simulink model "BigFourStEnCtrl"  (R2018b)
settings: Solver=FixedStepDiscrete  StartTime=0.0  StopTime=10.0  FixedStep=0.01  RelTol=1e-3
undefined symbols (not defined in the file or in its folder): data, KeSMSw4SSecRwLtStLgrstOtwdInwdClosePos1_Val, KeSMSw4SSecRwLtStLgrstUpwdDnwdClosePos1_Val, KeSMSw4SSecRwLtStLgrstUpwdDnwdClosePos2_Val, PassStBkReclnEn_Clear, PassStBkReclnEn_Set, PassStFwdBkwdEn_Clear, PassStFwdBkwdEn_Set, SecRwLtStBkReclnEn_Clear, SecRwLtStBkReclnEn_Set, SecRwLtStFwdBkwdEn_Clear, SecRwLtStFwdBkwdEn_Set, SecRwLtStLgrstInwdOtwdEn_Clear, SecRwLtStLgrstInwdOtwdEn_Set, SecRwLtStLgrstUpwdDnwdEn_Clear, SecRwLtStLgrstUpwdDnwdEn_Set, SecRwRtStBkReclnEn_Clear, SecRwRtStBkReclnEn_Set, SecRwRtStFwdBkwdEn_Clear, SecRwRtStFwdBkwdEn_Set, SecRwRtStLgrstInwdOtwdEn_Clear, SecRwRtStLgrstInwdOtwdEn_Set, SecRwRtStLgrstUpwdDnwdEn_Clear, SecRwRtStLgrstUpwdDnwdEn_Set, ThdRwLtStBkReclnEn_Clear, ThdRwLtStBkReclnEn_Set, ThdRwLtStCshnFldEn_Clear, ThdRwLtStCshnFldEn_Set, ThdRwLtStFwdBkwdEn_Clear, ThdRwLtStFwdBkwdEn_Set, ThdRwRtStBkReclnEn_Clear, ThdRwRtStBkReclnEn_Set, ThdRwRtStCshnFldEn_Clear, ThdRwRtStCshnFldEn_Set, ThdRwRtStFwdBkwdEn_Clear, ThdRwRtStFwdBkwdEn_Set, ZeroLEn_Clear, ZeroLEn_Set, ZeroREn_Clear, ZeroREn_Set
libraries: simulink x1
(part 1 of 2)
settings Model: Creator=sn2xws  LastModifiedBy=sn55gm
settings Model: ModifiedHistory=|
  | 2024.9.9 新增Md56
  | 2024.9.26 V3.0.1 从Md1V3.0.4复制
  | 2024.11.12 V3.0.2 Md1 bug 945653问题同步
settings DataIOCC: SaveFormat=StructureWithTime
settings OptimizationCC: DefaultParameterBehavior=Inlined  EnhancedBackFolding=on  PassReuseOutputArgsAs=Individual arguments  ZeroExternalMemoryAtStartup=off  ZeroInternalMemoryAtStartup=off  OptimizeBlockOrder=speed  DifferentSizesBufferReuse=on  OptimizationCustomize=off
settings DebuggingCC: ParameterTunabilityLossMsg=error
settings SFSimCC: MATLABDynamicMemAlloc=off
settings RTWCC: SystemTargetFile=autosar.tlc  GenCodeOnly=on  TemplateMakefile=ert_default_tmf  Description=AUTOSAR  GenerateReport=on  IncludeHyperlinkInReport=on  LaunchReport=on  GenerateTraceInfo=on  GenerateTraceReport=on  GenerateTraceReportSl=on  GenerateTraceReportSf=on  GenerateTraceReportEml=on
settings CodeAppCC: ForceParamTrailComments=on  IgnoreCustomStorageClasses=off  OperatorAnnotations=on  SimulinkDataObjDesc=on  SFDataObjDesc=on  InsertBlockDesc=on
settings STFCustomTargetCC: TargetLangStandard=C99 (ISO)  MultiwordLength=256  ParMdlRefBuildCompliant=on  CompOptLevelCompliant=on  IncludeMdlTerminateFcn=off  CombineOutputUpdateFcns=on  SuppressErrorStatus=on  ERTCustomFileBanners=on  SupportNonFinite=off  SupportComplex=off  SupportContinuousTime=off  SupportNonInlinedSFcns=off  RemoveResetFunc=on  MATLABClassNameForMDSCustomization=Simulink.SoftwareTarget.ERTCustomization  AutosarCompliant=on  UseToolchainInfoCompliant=on  LookupTableObjectStructAxisOrder=2,1,3,4,...  LUTObjectStructOrderEvenSpacing=Size,Table,Breakpoints  SystemTargetFile=autosar.tlc
settings ERTTargetCC: TargetLangStandard=C99 (ISO)  ConcurrentExecutionCompliant=off  IncludeMdlTerminateFcn=off  SuppressErrorStatus=on  SupportNonFinite=off  SupportComplex=off  ModelStepFunctionPrototypeControlCompliant=off  CPPClassGenCompliant=off  AutosarCompliant=on  LookupTableObjectStructAxisOrder=2,1,3,4,...  LUTObjectStructOrderEvenSpacing=Size,Table,Breakpoints  InlinedParameterPlacement=NonHierarchical  ERTCustomFileTemplate=example_file_process.tlc  ERTFilePackagingFormat=Compact  BooleanTrueId=TRUE  BooleanFalseId=FALSE

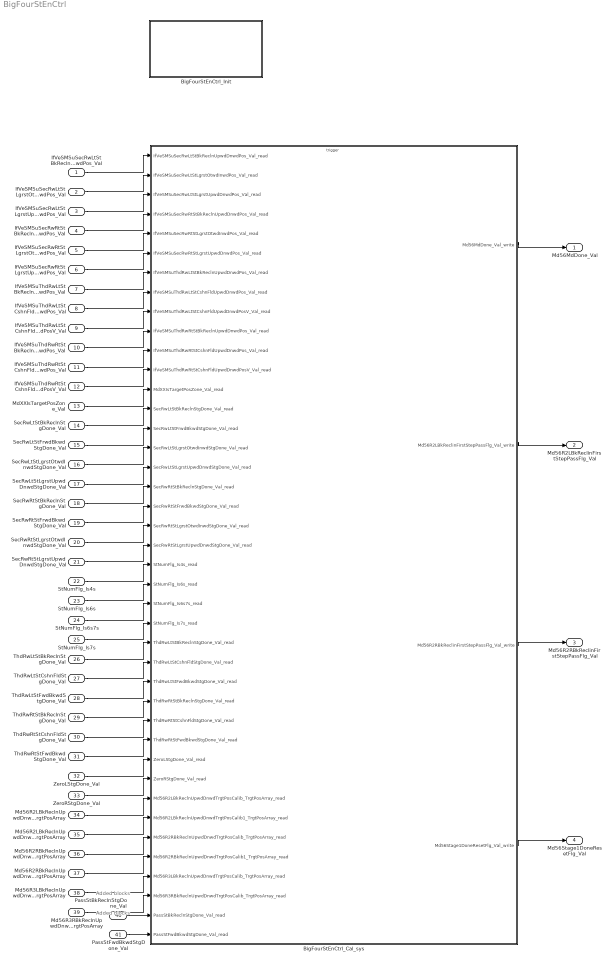
== system BigFourStEnCtrl ==
  note: Added blocks
  note: Added blocks
  IfVeSMSuSecRwLtStBkReclnUpwdDnwdPos_Val : Inport  OutDataTypeStr=uint16  PortDimensions=1
  IfVeSMSuSecRwLtStLgrstOtwdInwdPos_Val : Inport  Port=2  OutDataTypeStr=uint16  PortDimensions=1
  IfVeSMSuSecRwLtStLgrstUpwdDnwdPos_Val : Inport  Port=3  OutDataTypeStr=uint16  PortDimensions=1
  IfVeSMSuSecRwRtStBkReclnUpwdDnwdPos_Val : Inport  Port=4  OutDataTypeStr=uint16  PortDimensions=1
  IfVeSMSuSecRwRtStLgrstOtwdInwdPos_Val : Inport  Port=5  OutDataTypeStr=uint16  PortDimensions=1
  IfVeSMSuSecRwRtStLgrstUpwdDnwdPos_Val : Inport  Port=6  OutDataTypeStr=uint16  PortDimensions=1
  IfVeSMSuThdRwLtStBkReclnUpwdDnwdPos_Val : Inport  Port=7  OutDataTypeStr=uint16  PortDimensions=1
  IfVeSMSuThdRwLtStCshnFldUpwdDnwdPos_Val : Inport  Port=8  OutDataTypeStr=uint16  PortDimensions=1
  IfVeSMSuThdRwLtStCshnFldUpwdDnwdPosV_Val : Inport  Port=9  OutDataTypeStr=boolean  PortDimensions=1
  IfVeSMSuThdRwRtStBkReclnUpwdDnwdPos_Val : Inport  Port=10  OutDataTypeStr=uint16  PortDimensions=1
  IfVeSMSuThdRwRtStCshnFldUpwdDnwdPos_Val : Inport  Port=11  OutDataTypeStr=uint16  PortDimensions=1
  IfVeSMSuThdRwRtStCshnFldUpwdDnwdPosV_Val : Inport  Port=12  OutDataTypeStr=boolean  PortDimensions=1
  MdXXIsTargetPosZone_Val : Inport  Port=13  OutDataTypeStr=uint32  PortDimensions=1
  SecRwLtStBkReclnStgDone_Val : Inport  Port=14  OutDataTypeStr=boolean  PortDimensions=1
  SecRwLtStFrwdBkwdStgDone_Val : Inport  Port=15  OutDataTypeStr=boolean  PortDimensions=1
  SecRwLtStLgrstOtwdInwdStgDone_Val : Inport  Port=16  OutDataTypeStr=boolean  PortDimensions=1
  SecRwLtStLgrstUpwdDnwdStgDone_Val : Inport  Port=17  OutDataTypeStr=boolean  PortDimensions=1
  SecRwRtStBkReclnStgDone_Val : Inport  Port=18  OutDataTypeStr=boolean  PortDimensions=1
  SecRwRtStFrwdBkwdStgDone_Val : Inport  Port=19  OutDataTypeStr=boolean  PortDimensions=1
  SecRwRtStLgrstOtwdInwdStgDone_Val : Inport  Port=20  OutDataTypeStr=boolean  PortDimensions=1
  SecRwRtStLgrstUpwdDnwdStgDone_Val : Inport  Port=21  OutDataTypeStr=boolean  PortDimensions=1
  StNumFlg_Is4s : Inport  Port=22  OutDataTypeStr=boolean  PortDimensions=1
  StNumFlg_Is6s : Inport  Port=23  OutDataTypeStr=boolean  PortDimensions=1
  StNumFlg_Is6s7s : Inport  Port=24  OutDataTypeStr=boolean  PortDimensions=1
  StNumFlg_Is7s : Inport  Port=25  OutDataTypeStr=boolean  PortDimensions=1
  ThdRwLtStBkReclnStgDone_Val : Inport  Port=26  OutDataTypeStr=boolean  PortDimensions=1
  ThdRwLtStCshnFldStgDone_Val : Inport  Port=27  OutDataTypeStr=boolean  PortDimensions=1
  ThdRwLtStFwdBkwdStgDone_Val : Inport  Port=28  OutDataTypeStr=boolean  PortDimensions=1
  ThdRwRtStBkReclnStgDone_Val : Inport  Port=29  OutDataTypeStr=boolean  PortDimensions=1
  ThdRwRtStCshnFldStgDone_Val : Inport  Port=30  OutDataTypeStr=boolean  PortDimensions=1
  ThdRwRtStFwdBkwdStgDone_Val : Inport  Port=31  OutDataTypeStr=boolean  PortDimensions=1
  ZeroLStgDone_Val : Inport  Port=32  OutDataTypeStr=boolean  PortDimensions=1
  ZeroRStgDone_Val : Inport  Port=33  OutDataTypeStr=boolean  PortDimensions=1
  Md56R2LBkReclnUpwdDnwdTrgtPosCalib_TrgtPosArray : Inport  Description=|  Port=34  OutDataTypeStr=uint16  PortDimensions=3
      | 0:Pos
      | 1:Max
      | 2:Min
  Md56R2LBkReclnUpwdDnwdTrgtPosCalib1_TrgtPosArray : Inport  Description=|  Port=35  OutDataTypeStr=uint16  PortDimensions=3
      | 0:Pos
      | 1:Max
      | 2:Min
  Md56R2RBkReclnUpwdDnwdTrgtPosCalib_TrgtPosArray : Inport  Description=|  Port=36  OutDataTypeStr=uint16  PortDimensions=3
      | 0:Pos
      | 1:Max
      | 2:Min
  Md56R2RBkReclnUpwdDnwdTrgtPosCalib1_TrgtPosArray : Inport  Description=|  Port=37  OutDataTypeStr=uint16  PortDimensions=3
      | 0:Pos
      | 1:Max
      | 2:Min
  Md56R3LBkReclnUpwdDnwdTrgtPosCalib_TrgtPosArray : Inport  Description=|  Port=38  OutDataTypeStr=uint16  PortDimensions=3
      | 0:Pos
      | 1:Max
      | 2:Min
  Md56R3RBkReclnUpwdDnwdTrgtPosCalib_TrgtPosArray : Inport  Description=|  Port=39  OutDataTypeStr=uint16  PortDimensions=3
      | 0:Pos
      | 1:Max
      | 2:Min
  PassStBkReclnStgDone_Val : Inport  Port=40  OutDataTypeStr=boolean  PortDimensions=1
  PassStFwdBkwdStgDone_Val : Inport  Port=41  OutDataTypeStr=boolean  PortDimensions=1
  BigFourStEnCtrl_Cal_sys : Subsystem
  BigFourStEnCtrl_Init : Subsystem
  Md56MdDone_Val : Outport  OutDataTypeStr=uint8  PortDimensions=1
  Md56R2LBkReclinFirstStepPassFlg_Val : Outport  Port=2  OutDataTypeStr=boolean  PortDimensions=1
  Md56R2RBkReclinFirstStepPassFlg_Val : Outport  Port=3  OutDataTypeStr=boolean  PortDimensions=1
  Md56Stage1DoneResetFlg_Val : Outport  Port=4  OutDataTypeStr=boolean  PortDimensions=1
  wires:
  IfVeSMSuSecRwLtStBkReclnUpwdDnwdPos_Val/1 -> BigFourStEnCtrl_Cal_sys/1(IfVeSMSuSecRwLtStBkReclnUpwdDnwdPos_Val_read)
  IfVeSMSuSecRwLtStLgrstOtwdInwdPos_Val/1 -> BigFourStEnCtrl_Cal_sys/2(IfVeSMSuSecRwLtStLgrstOtwdInwdPos_Val_read)
  IfVeSMSuSecRwLtStLgrstUpwdDnwdPos_Val/1 -> BigFourStEnCtrl_Cal_sys/3(IfVeSMSuSecRwLtStLgrstUpwdDnwdPos_Val_read)
  IfVeSMSuSecRwRtStBkReclnUpwdDnwdPos_Val/1 -> BigFourStEnCtrl_Cal_sys/4(IfVeSMSuSecRwRtStBkReclnUpwdDnwdPos_Val_read)
  IfVeSMSuSecRwRtStLgrstOtwdInwdPos_Val/1 -> BigFourStEnCtrl_Cal_sys/5(IfVeSMSuSecRwRtStLgrstOtwdInwdPos_Val_read)
  IfVeSMSuSecRwRtStLgrstUpwdDnwdPos_Val/1 -> BigFourStEnCtrl_Cal_sys/6(IfVeSMSuSecRwRtStLgrstUpwdDnwdPos_Val_read)
  IfVeSMSuThdRwLtStBkReclnUpwdDnwdPos_Val/1 -> BigFourStEnCtrl_Cal_sys/7(IfVeSMSuThdRwLtStBkReclnUpwdDnwdPos_Val_read)
  IfVeSMSuThdRwLtStCshnFldUpwdDnwdPos_Val/1 -> BigFourStEnCtrl_Cal_sys/8(IfVeSMSuThdRwLtStCshnFldUpwdDnwdPos_Val_read)
  IfVeSMSuThdRwLtStCshnFldUpwdDnwdPosV_Val/1 -> BigFourStEnCtrl_Cal_sys/9(IfVeSMSuThdRwLtStCshnFldUpwdDnwdPosV_Val_read)
  IfVeSMSuThdRwRtStBkReclnUpwdDnwdPos_Val/1 -> BigFourStEnCtrl_Cal_sys/10(IfVeSMSuThdRwRtStBkReclnUpwdDnwdPos_Val_read)
  IfVeSMSuThdRwRtStCshnFldUpwdDnwdPos_Val/1 -> BigFourStEnCtrl_Cal_sys/11(IfVeSMSuThdRwRtStCshnFldUpwdDnwdPos_Val_read)
  IfVeSMSuThdRwRtStCshnFldUpwdDnwdPosV_Val/1 -> BigFourStEnCtrl_Cal_sys/12(IfVeSMSuThdRwRtStCshnFldUpwdDnwdPosV_Val_read)
  MdXXIsTargetPosZone_Val/1 -> BigFourStEnCtrl_Cal_sys/13(MdXXIsTargetPosZone_Val_read)
  SecRwLtStBkReclnStgDone_Val/1 -> BigFourStEnCtrl_Cal_sys/14(SecRwLtStBkReclnStgDone_Val_read)
  SecRwLtStFrwdBkwdStgDone_Val/1 -> BigFourStEnCtrl_Cal_sys/15(SecRwLtStFrwdBkwdStgDone_Val_read)
  SecRwLtStLgrstOtwdInwdStgDone_Val/1 -> BigFourStEnCtrl_Cal_sys/16(SecRwLtStLgrstOtwdInwdStgDone_Val_read)
  SecRwLtStLgrstUpwdDnwdStgDone_Val/1 -> BigFourStEnCtrl_Cal_sys/17(SecRwLtStLgrstUpwdDnwdStgDone_Val_read)
  SecRwRtStBkReclnStgDone_Val/1 -> BigFourStEnCtrl_Cal_sys/18(SecRwRtStBkReclnStgDone_Val_read)
  SecRwRtStFrwdBkwdStgDone_Val/1 -> BigFourStEnCtrl_Cal_sys/19(SecRwRtStFrwdBkwdStgDone_Val_read)
  SecRwRtStLgrstOtwdInwdStgDone_Val/1 -> BigFourStEnCtrl_Cal_sys/20(SecRwRtStLgrstOtwdInwdStgDone_Val_read)
  SecRwRtStLgrstUpwdDnwdStgDone_Val/1 -> BigFourStEnCtrl_Cal_sys/21(SecRwRtStLgrstUpwdDnwdStgDone_Val_read)
  StNumFlg_Is4s/1 -> BigFourStEnCtrl_Cal_sys/22(StNumFlg_Is4s_read)
  StNumFlg_Is6s/1 -> BigFourStEnCtrl_Cal_sys/23(StNumFlg_Is6s_read)
  StNumFlg_Is6s7s/1 -> BigFourStEnCtrl_Cal_sys/24(StNumFlg_Is6s7s_read)
  StNumFlg_Is7s/1 -> BigFourStEnCtrl_Cal_sys/25(StNumFlg_Is7s_read)
  ThdRwLtStBkReclnStgDone_Val/1 -> BigFourStEnCtrl_Cal_sys/26(ThdRwLtStBkReclnStgDone_Val_read)
  ThdRwLtStCshnFldStgDone_Val/1 -> BigFourStEnCtrl_Cal_sys/27(ThdRwLtStCshnFldStgDone_Val_read)
  ThdRwLtStFwdBkwdStgDone_Val/1 -> BigFourStEnCtrl_Cal_sys/28(ThdRwLtStFwdBkwdStgDone_Val_read)
  ThdRwRtStBkReclnStgDone_Val/1 -> BigFourStEnCtrl_Cal_sys/29(ThdRwRtStBkReclnStgDone_Val_read)
  ThdRwRtStCshnFldStgDone_Val/1 -> BigFourStEnCtrl_Cal_sys/30(ThdRwRtStCshnFldStgDone_Val_read)
  ThdRwRtStFwdBkwdStgDone_Val/1 -> BigFourStEnCtrl_Cal_sys/31(ThdRwRtStFwdBkwdStgDone_Val_read)
  ZeroLStgDone_Val/1 -> BigFourStEnCtrl_Cal_sys/32(ZeroLStgDone_Val_read)
  ZeroRStgDone_Val/1 -> BigFourStEnCtrl_Cal_sys/33(ZeroRStgDone_Val_read)
  Md56R2LBkReclnUpwdDnwdTrgtPosCalib_TrgtPosArray/1 -> BigFourStEnCtrl_Cal_sys/34(Md56R2LBkReclnUpwdDnwdTrgtPosCalib_TrgtPosArray_read)
  Md56R2LBkReclnUpwdDnwdTrgtPosCalib1_TrgtPosArray/1 -> BigFourStEnCtrl_Cal_sys/35(Md56R2LBkReclnUpwdDnwdTrgtPosCalib1_TrgtPosArray_read)
  Md56R2RBkReclnUpwdDnwdTrgtPosCalib_TrgtPosArray/1 -> BigFourStEnCtrl_Cal_sys/36(Md56R2RBkReclnUpwdDnwdTrgtPosCalib_TrgtPosArray_read)
  Md56R2RBkReclnUpwdDnwdTrgtPosCalib1_TrgtPosArray/1 -> BigFourStEnCtrl_Cal_sys/37(Md56R2RBkReclnUpwdDnwdTrgtPosCalib1_TrgtPosArray_read)
  Md56R3LBkReclnUpwdDnwdTrgtPosCalib_TrgtPosArray/1 -> BigFourStEnCtrl_Cal_sys/38(Md56R3LBkReclnUpwdDnwdTrgtPosCalib_TrgtPosArray_read)
  Md56R3RBkReclnUpwdDnwdTrgtPosCalib_TrgtPosArray/1 -> BigFourStEnCtrl_Cal_sys/39(Md56R3RBkReclnUpwdDnwdTrgtPosCalib_TrgtPosArray_read)
  BigFourStEnCtrl_Cal_sys/1(Md56MdDone_Val_write) -> Md56MdDone_Val/1
  BigFourStEnCtrl_Cal_sys/2(Md56R2LBkReclinFirstStepPassFlg_Val_write) -> Md56R2LBkReclinFirstStepPassFlg_Val/1
  BigFourStEnCtrl_Cal_sys/3(Md56R2RBkReclinFirstStepPassFlg_Val_write) -> Md56R2RBkReclinFirstStepPassFlg_Val/1
  BigFourStEnCtrl_Cal_sys/4(Md56Stage1DoneResetFlg_Val_write) -> Md56Stage1DoneResetFlg_Val/1
  PassStBkReclnStgDone_Val/1 -> BigFourStEnCtrl_Cal_sys/40(PassStBkReclnStgDone_Val_read)
  PassStFwdBkwdStgDone_Val/1 -> BigFourStEnCtrl_Cal_sys/41(PassStFwdBkwdStgDone_Val_read)

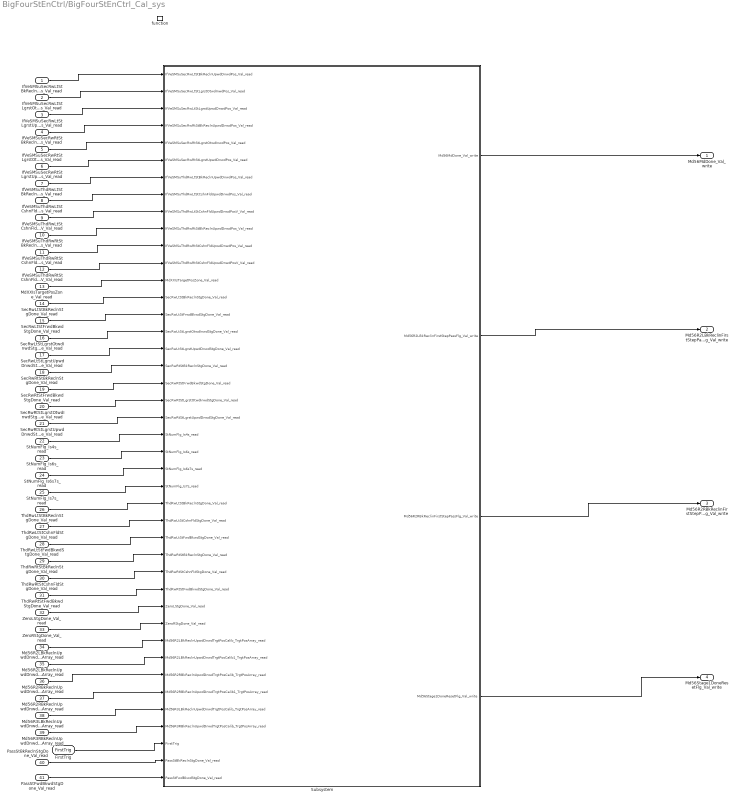
== system BigFourStEnCtrl/BigFourStEnCtrl_Cal_sys ==
  IfVeSMSuSecRwLtStBkReclnUpwdDnwdPos_Val_read : Inport
  IfVeSMSuSecRwLtStLgrstOtwdInwdPos_Val_read : Inport  Port=2
  IfVeSMSuSecRwLtStLgrstUpwdDnwdPos_Val_read : Inport  Port=3
  IfVeSMSuSecRwRtStBkReclnUpwdDnwdPos_Val_read : Inport  Port=4
  IfVeSMSuSecRwRtStLgrstOtwdInwdPos_Val_read : Inport  Port=5
  IfVeSMSuSecRwRtStLgrstUpwdDnwdPos_Val_read : Inport  Port=6
  IfVeSMSuThdRwLtStBkReclnUpwdDnwdPos_Val_read : Inport  Port=7
  IfVeSMSuThdRwLtStCshnFldUpwdDnwdPos_Val_read : Inport  Port=8
  IfVeSMSuThdRwLtStCshnFldUpwdDnwdPosV_Val_read : Inport  Port=9
  IfVeSMSuThdRwRtStBkReclnUpwdDnwdPos_Val_read : Inport  Port=10
  IfVeSMSuThdRwRtStCshnFldUpwdDnwdPos_Val_read : Inport  Port=11
  IfVeSMSuThdRwRtStCshnFldUpwdDnwdPosV_Val_read : Inport  Port=12
  MdXXIsTargetPosZone_Val_read : Inport  Port=13
  SecRwLtStBkReclnStgDone_Val_read : Inport  Port=14
  SecRwLtStFrwdBkwdStgDone_Val_read : Inport  Port=15
  SecRwLtStLgrstOtwdInwdStgDone_Val_read : Inport  Port=16
  SecRwLtStLgrstUpwdDnwdStgDone_Val_read : Inport  Port=17
  SecRwRtStBkReclnStgDone_Val_read : Inport  Port=18
  SecRwRtStFrwdBkwdStgDone_Val_read : Inport  Port=19
  SecRwRtStLgrstOtwdInwdStgDone_Val_read : Inport  Port=20
  SecRwRtStLgrstUpwdDnwdStgDone_Val_read : Inport  Port=21
  StNumFlg_Is4s_read : Inport  Port=22
  StNumFlg_Is6s_read : Inport  Port=23
  StNumFlg_Is6s7s_read : Inport  Port=24
  StNumFlg_Is7s_read : Inport  Port=25
  ThdRwLtStBkReclnStgDone_Val_read : Inport  Port=26
  ThdRwLtStCshnFldStgDone_Val_read : Inport  Port=27
  ThdRwLtStFwdBkwdStgDone_Val_read : Inport  Port=28
  ThdRwRtStBkReclnStgDone_Val_read : Inport  Port=29
  ThdRwRtStCshnFldStgDone_Val_read : Inport  Port=30
  ThdRwRtStFwdBkwdStgDone_Val_read : Inport  Port=31
  ZeroLStgDone_Val_read : Inport  Port=32
  ZeroRStgDone_Val_read : Inport  Port=33
  Md56R2LBkReclnUpwdDnwdTrgtPosCalib_TrgtPosArray_read : Inport  Port=34
  Md56R2LBkReclnUpwdDnwdTrgtPosCalib1_TrgtPosArray_read : Inport  Port=35
  Md56R2RBkReclnUpwdDnwdTrgtPosCalib_TrgtPosArray_read : Inport  Port=36
  Md56R2RBkReclnUpwdDnwdTrgtPosCalib1_TrgtPosArray_read : Inport  Port=37
  Md56R3LBkReclnUpwdDnwdTrgtPosCalib_TrgtPosArray_read : Inport  Port=38
  Md56R3RBkReclnUpwdDnwdTrgtPosCalib_TrgtPosArray_read : Inport  Port=39
  PassStBkReclnStgDone_Val_read : Inport  Port=40
  PassStFwdBkwdStgDone_Val_read : Inport  Port=41
  function : TriggerPort  TriggerType=function-call  IsSimulinkFunction=on  FunctionName=BigFourStEnCtrl_Cal  VariantControl=(inherit)
  Subsystem : Subsystem
  FirstTrig : ArgIn  OutDataTypeStr=boolean  ArgumentName=FirstTrig
  Md56MdDone_Val_write : Outport
      settings: EnsureOutportIsVirtual=on
  Md56R2LBkReclinFirstStepPassFlg_Val_write : Outport  Port=2
      settings: EnsureOutportIsVirtual=on
  Md56R2RBkReclinFirstStepPassFlg_Val_write : Outport  Port=3
      settings: EnsureOutportIsVirtual=on
  Md56Stage1DoneResetFlg_Val_write : Outport  Port=4
      settings: EnsureOutportIsVirtual=on
  wires:
  IfVeSMSuSecRwLtStBkReclnUpwdDnwdPos_Val_read/1 -> Subsystem/1(IfVeSMSuSecRwLtStBkReclnUpwdDnwdPos_Val_read)
  IfVeSMSuSecRwLtStLgrstOtwdInwdPos_Val_read/1 -> Subsystem/2(IfVeSMSuSecRwLtStLgrstOtwdInwdPos_Val_read)
  IfVeSMSuSecRwLtStLgrstUpwdDnwdPos_Val_read/1 -> Subsystem/3(IfVeSMSuSecRwLtStLgrstUpwdDnwdPos_Val_read)
  IfVeSMSuSecRwRtStBkReclnUpwdDnwdPos_Val_read/1 -> Subsystem/4(IfVeSMSuSecRwRtStBkReclnUpwdDnwdPos_Val_read)
  IfVeSMSuSecRwRtStLgrstOtwdInwdPos_Val_read/1 -> Subsystem/5(IfVeSMSuSecRwRtStLgrstOtwdInwdPos_Val_read)
  IfVeSMSuSecRwRtStLgrstUpwdDnwdPos_Val_read/1 -> Subsystem/6(IfVeSMSuSecRwRtStLgrstUpwdDnwdPos_Val_read)
  IfVeSMSuThdRwLtStBkReclnUpwdDnwdPos_Val_read/1 -> Subsystem/7(IfVeSMSuThdRwLtStBkReclnUpwdDnwdPos_Val_read)
  IfVeSMSuThdRwLtStCshnFldUpwdDnwdPos_Val_read/1 -> Subsystem/8(IfVeSMSuThdRwLtStCshnFldUpwdDnwdPos_Val_read)
  IfVeSMSuThdRwLtStCshnFldUpwdDnwdPosV_Val_read/1 -> Subsystem/9(IfVeSMSuThdRwLtStCshnFldUpwdDnwdPosV_Val_read)
  IfVeSMSuThdRwRtStBkReclnUpwdDnwdPos_Val_read/1 -> Subsystem/10(IfVeSMSuThdRwRtStBkReclnUpwdDnwdPos_Val_read)
  IfVeSMSuThdRwRtStCshnFldUpwdDnwdPos_Val_read/1 -> Subsystem/11(IfVeSMSuThdRwRtStCshnFldUpwdDnwdPos_Val_read)
  IfVeSMSuThdRwRtStCshnFldUpwdDnwdPosV_Val_read/1 -> Subsystem/12(IfVeSMSuThdRwRtStCshnFldUpwdDnwdPosV_Val_read)
  MdXXIsTargetPosZone_Val_read/1 -> Subsystem/13(MdXXIsTargetPosZone_Val_read)
  SecRwLtStBkReclnStgDone_Val_read/1 -> Subsystem/14(SecRwLtStBkReclnStgDone_Val_read)
  SecRwLtStFrwdBkwdStgDone_Val_read/1 -> Subsystem/15(SecRwLtStFrwdBkwdStgDone_Val_read)
  SecRwLtStLgrstOtwdInwdStgDone_Val_read/1 -> Subsystem/16(SecRwLtStLgrstOtwdInwdStgDone_Val_read)
  SecRwLtStLgrstUpwdDnwdStgDone_Val_read/1 -> Subsystem/17(SecRwLtStLgrstUpwdDnwdStgDone_Val_read)
  SecRwRtStBkReclnStgDone_Val_read/1 -> Subsystem/18(SecRwRtStBkReclnStgDone_Val_read)
  SecRwRtStFrwdBkwdStgDone_Val_read/1 -> Subsystem/19(SecRwRtStFrwdBkwdStgDone_Val_read)
  SecRwRtStLgrstOtwdInwdStgDone_Val_read/1 -> Subsystem/20(SecRwRtStLgrstOtwdInwdStgDone_Val_read)
  SecRwRtStLgrstUpwdDnwdStgDone_Val_read/1 -> Subsystem/21(SecRwRtStLgrstUpwdDnwdStgDone_Val_read)
  StNumFlg_Is4s_read/1 -> Subsystem/22(StNumFlg_Is4s_read)
  StNumFlg_Is6s_read/1 -> Subsystem/23(StNumFlg_Is6s_read)
  StNumFlg_Is6s7s_read/1 -> Subsystem/24(StNumFlg_Is6s7s_read)
  StNumFlg_Is7s_read/1 -> Subsystem/25(StNumFlg_Is7s_read)
  ThdRwLtStBkReclnStgDone_Val_read/1 -> Subsystem/26(ThdRwLtStBkReclnStgDone_Val_read)
  ThdRwLtStCshnFldStgDone_Val_read/1 -> Subsystem/27(ThdRwLtStCshnFldStgDone_Val_read)
  ThdRwLtStFwdBkwdStgDone_Val_read/1 -> Subsystem/28(ThdRwLtStFwdBkwdStgDone_Val_read)
  ThdRwRtStBkReclnStgDone_Val_read/1 -> Subsystem/29(ThdRwRtStBkReclnStgDone_Val_read)
  ThdRwRtStCshnFldStgDone_Val_read/1 -> Subsystem/30(ThdRwRtStCshnFldStgDone_Val_read)
  ThdRwRtStFwdBkwdStgDone_Val_read/1 -> Subsystem/31(ThdRwRtStFwdBkwdStgDone_Val_read)
  ZeroLStgDone_Val_read/1 -> Subsystem/32(ZeroLStgDone_Val_read)
  ZeroRStgDone_Val_read/1 -> Subsystem/33(ZeroRStgDone_Val_read)
  Md56R2LBkReclnUpwdDnwdTrgtPosCalib_TrgtPosArray_read/1 -> Subsystem/34(Md56R2LBkReclnUpwdDnwdTrgtPosCalib_TrgtPosArray_read)
  Md56R2LBkReclnUpwdDnwdTrgtPosCalib1_TrgtPosArray_read/1 -> Subsystem/35(Md56R2LBkReclnUpwdDnwdTrgtPosCalib1_TrgtPosArray_read)
  Md56R2RBkReclnUpwdDnwdTrgtPosCalib_TrgtPosArray_read/1 -> Subsystem/36(Md56R2RBkReclnUpwdDnwdTrgtPosCalib_TrgtPosArray_read)
  Md56R2RBkReclnUpwdDnwdTrgtPosCalib1_TrgtPosArray_read/1 -> Subsystem/37(Md56R2RBkReclnUpwdDnwdTrgtPosCalib1_TrgtPosArray_read)
  Md56R3LBkReclnUpwdDnwdTrgtPosCalib_TrgtPosArray_read/1 -> Subsystem/38(Md56R3LBkReclnUpwdDnwdTrgtPosCalib_TrgtPosArray_read)
  Md56R3RBkReclnUpwdDnwdTrgtPosCalib_TrgtPosArray_read/1 -> Subsystem/39(Md56R3RBkReclnUpwdDnwdTrgtPosCalib_TrgtPosArray_read)
  FirstTrig/1 -> Subsystem/40(FirstTrig)
  Subsystem/1(Md56MdDone_Val_write) -> Md56MdDone_Val_write/1
  Subsystem/2(Md56R2LBkReclinFirstStepPassFlg_Val_write) -> Md56R2LBkReclinFirstStepPassFlg_Val_write/1
  Subsystem/3(Md56R2RBkReclinFirstStepPassFlg_Val_write) -> Md56R2RBkReclinFirstStepPassFlg_Val_write/1
  Subsystem/4(Md56Stage1DoneResetFlg_Val_write) -> Md56Stage1DoneResetFlg_Val_write/1
  PassStBkReclnStgDone_Val_read/1 -> Subsystem/41(PassStBkReclnStgDone_Val_read)
  PassStFwdBkwdStgDone_Val_read/1 -> Subsystem/42(PassStFwdBkwdStgDone_Val_read)

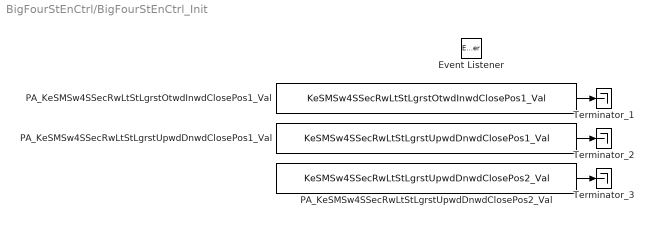
== system BigFourStEnCtrl/BigFourStEnCtrl_Init ==
  Event Listener : EventListener  EventName=reset
  PA_KeSMSw4SSecRwLtStLgrstOtwdInwdClosePos1_Val : Constant  Value=KeSMSw4SSecRwLtStLgrstOtwdInwdClosePos1_Val
  PA_KeSMSw4SSecRwLtStLgrstUpwdDnwdClosePos1_Val : Constant  Value=KeSMSw4SSecRwLtStLgrstUpwdDnwdClosePos1_Val
  PA_KeSMSw4SSecRwLtStLgrstUpwdDnwdClosePos2_Val : Constant  Value=KeSMSw4SSecRwLtStLgrstUpwdDnwdClosePos2_Val
  Terminator_1 : Terminator
  Terminator_2 : Terminator
  Terminator_3 : Terminator
  wires:
  PA_KeSMSw4SSecRwLtStLgrstOtwdInwdClosePos1_Val/1 -> Terminator_1/1
  PA_KeSMSw4SSecRwLtStLgrstUpwdDnwdClosePos1_Val/1 -> Terminator_2/1
  PA_KeSMSw4SSecRwLtStLgrstUpwdDnwdClosePos2_Val/1 -> Terminator_3/1

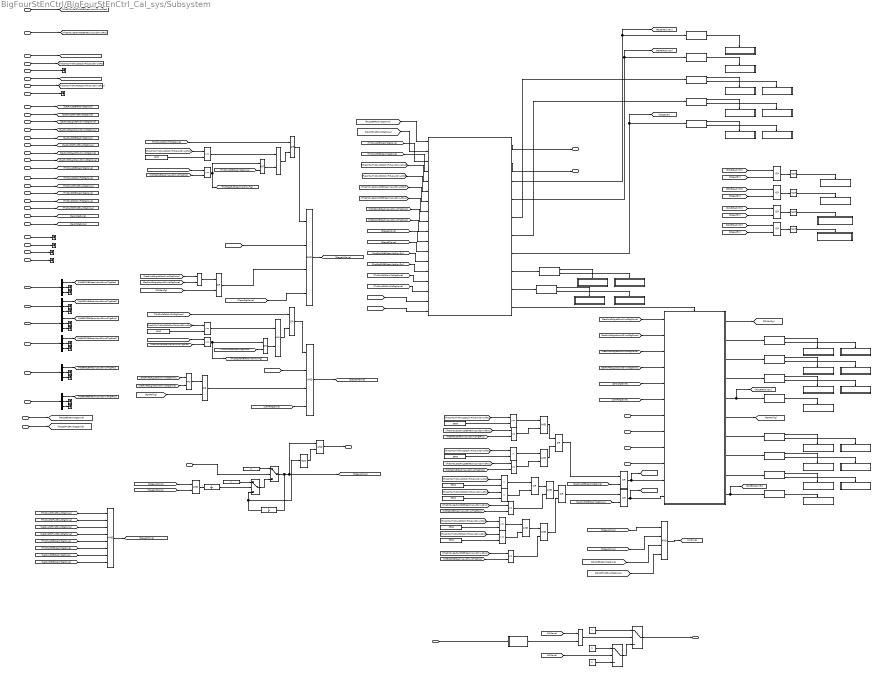
== system BigFourStEnCtrl/BigFourStEnCtrl_Cal_sys/Subsystem ==
  IfVeSMSuSecRwLtStBkReclnUpwdDnwdPos_Val_read : Inport
  IfVeSMSuSecRwLtStLgrstOtwdInwdPos_Val_read : Inport  Port=2
  IfVeSMSuSecRwLtStLgrstUpwdDnwdPos_Val_read : Inport  Port=3
  IfVeSMSuSecRwRtStBkReclnUpwdDnwdPos_Val_read : Inport  Port=4
  IfVeSMSuSecRwRtStLgrstOtwdInwdPos_Val_read : Inport  Port=5
  IfVeSMSuSecRwRtStLgrstUpwdDnwdPos_Val_read : Inport  Port=6
  IfVeSMSuThdRwLtStBkReclnUpwdDnwdPos_Val_read : Inport  Port=7
  IfVeSMSuThdRwLtStCshnFldUpwdDnwdPos_Val_read : Inport  Port=8
  IfVeSMSuThdRwLtStCshnFldUpwdDnwdPosV_Val_read : Inport  Port=9
  IfVeSMSuThdRwRtStBkReclnUpwdDnwdPos_Val_read : Inport  Port=10
  IfVeSMSuThdRwRtStCshnFldUpwdDnwdPos_Val_read : Inport  Port=11
  IfVeSMSuThdRwRtStCshnFldUpwdDnwdPosV_Val_read : Inport  Port=12
  MdXXIsTargetPosZone_Val_read : Inport  Port=13
  SecRwLtStBkReclnStgDone_Val_read : Inport  Port=14
  SecRwLtStFrwdBkwdStgDone_Val_read : Inport  Port=15
  SecRwLtStLgrstOtwdInwdStgDone_Val_read : Inport  Port=16
  SecRwLtStLgrstUpwdDnwdStgDone_Val_read : Inport  Port=17
  SecRwRtStBkReclnStgDone_Val_read : Inport  Port=18
  SecRwRtStFrwdBkwdStgDone_Val_read : Inport  Port=19
  SecRwRtStLgrstOtwdInwdStgDone_Val_read : Inport  Port=20
  SecRwRtStLgrstUpwdDnwdStgDone_Val_read : Inport  Port=21
  StNumFlg_Is4s_read : Inport  Port=22
  StNumFlg_Is6s_read : Inport  Port=23
  StNumFlg_Is6s7s_read : Inport  Port=24
  StNumFlg_Is7s_read : Inport  Port=25
  ThdRwLtStBkReclnStgDone_Val_read : Inport  Port=26
  ThdRwLtStCshnFldStgDone_Val_read : Inport  Port=27
  ThdRwLtStFwdBkwdStgDone_Val_read : Inport  Port=28
  ThdRwRtStBkReclnStgDone_Val_read : Inport  Port=29
  ThdRwRtStCshnFldStgDone_Val_read : Inport  Port=30
  ThdRwRtStFwdBkwdStgDone_Val_read : Inport  Port=31
  ZeroLStgDone_Val_read : Inport  Port=32
  ZeroRStgDone_Val_read : Inport  Port=33
  Md56R2LBkReclnUpwdDnwdTrgtPosCalib_TrgtPosArray_read : Inport  Port=34
  Md56R2LBkReclnUpwdDnwdTrgtPosCalib1_TrgtPosArray_read : Inport  Port=35
  Md56R2RBkReclnUpwdDnwdTrgtPosCalib_TrgtPosArray_read : Inport  Port=36
  Md56R2RBkReclnUpwdDnwdTrgtPosCalib1_TrgtPosArray_read : Inport  Port=37
  Md56R3LBkReclnUpwdDnwdTrgtPosCalib_TrgtPosArray_read : Inport  Port=38
  Md56R3RBkReclnUpwdDnwdTrgtPosCalib_TrgtPosArray_read : Inport  Port=39
  FirstTrig : Inport  Port=40
  PassStBkReclnStgDone_Val_read : Inport  Port=41
  PassStFwdBkwdStgDone_Val_read : Inport  Port=42
  32BitSelector : Subsystem  mask(32 Bit Selector){BitNum=24}
      mask prompts: BitNum "Select Bit Number"
      mask help: Allows selection of a particular bit (0-31) out of a packed word up to 32 bits long. Output will be true if the bit number selected via the mask parameter is equal to one.
      mask TypeOptions BitNum: 0 | 1 | 2 | 3 | 4 | 5 | 6 | 7 | 8 | 9 | 10 | 11 | 12 | 13 | 14 | 15 | 16 | 17 | 18 | 19 | 20 | 21 | 22 | 23 | 24 | 25 | 26 | 27 | 28 | 29 | 30 | 31
      mask Display:
      | text(0.5, 0.8,'BIT','horizontalAlignment','center')
      | text(0.5, 0.5,'SELECTOR','horizontalAlignment','center')
      | text(0.5, 0.2,['-- Bit ',char(get_param(gcb,'BitNum')),' --'],'horizontalAlignment','center')
  Chart : Stateflow chart  TreatAsAtomicUnit=on
  Constant : Constant  OutDataTypeStr=uint8
  Constant1 : Constant  Value=2  OutDataTypeStr=uint8
  Constant{7..9,11..13} (6 alike) : Constant  Value=3960  OutDataTypeStr=uint16  SampleTime=-1
  Constant2 : Constant  Value=0  OutDataTypeStr=uint8
  Constant3 : Constant  Value=4000  OutDataTypeStr=uint16  SampleTime=-1
  Constant4 : Constant  Value=4000  OutDataTypeStr=uint16  SampleTime=-1
  Constant5 : Constant  Value=0
  Constant6 : Constant
  Demux{1..6} (6 alike) : Demux  Outputs=3
  If Action Subsystem1 : Subsystem  TreatAsAtomicUnit=on
  If Action Subsystem10 : Subsystem  TreatAsAtomicUnit=on
  If Action Subsystem11 : Subsystem  TreatAsAtomicUnit=on
  If Action Subsystem12 : Subsystem  TreatAsAtomicUnit=on
  If Action Subsystem13 : Subsystem  TreatAsAtomicUnit=on
  If Action Subsystem14 : Subsystem  TreatAsAtomicUnit=on
  If Action Subsystem15 : Subsystem  TreatAsAtomicUnit=on
  If Action Subsystem16 : Subsystem  TreatAsAtomicUnit=on
  If Action Subsystem17 : Subsystem  TreatAsAtomicUnit=on
  If Action Subsystem18 : Subsystem  TreatAsAtomicUnit=on
  If Action Subsystem19 : Subsystem  TreatAsAtomicUnit=on
  If Action Subsystem2 : Subsystem  TreatAsAtomicUnit=on
  If Action Subsystem20 : Subsystem  TreatAsAtomicUnit=on
  If Action Subsystem21 : Subsystem  TreatAsAtomicUnit=on
  If Action Subsystem22 : Subsystem  TreatAsAtomicUnit=on
  If Action Subsystem23 : Subsystem  TreatAsAtomicUnit=on
  If Action Subsystem24 : Subsystem  TreatAsAtomicUnit=on
  If Action Subsystem25 : Subsystem  TreatAsAtomicUnit=on
  If Action Subsystem26 : Subsystem  TreatAsAtomicUnit=on
  If Action Subsystem27 : Subsystem  TreatAsAtomicUnit=on
  If Action Subsystem28 : Subsystem  TreatAsAtomicUnit=on
  If Action Subsystem3 : Subsystem  TreatAsAtomicUnit=on
  If Action Subsystem4 : Subsystem  TreatAsAtomicUnit=on
  If Action Subsystem5 : Subsystem  TreatAsAtomicUnit=on
  If Action Subsystem6 : Subsystem  TreatAsAtomicUnit=on
  If Action Subsystem7 : Subsystem  TreatAsAtomicUnit=on
  If Action Subsystem8 : Subsystem  TreatAsAtomicUnit=on
  If Action Subsystem9 : Subsystem  TreatAsAtomicUnit=on
  If{1,6,14..15} (4 alike) : If  IfExpression=u1  ShowElse=off
  If{2..5,7..13} (11 alike) : If  IfExpression=u1
  Logical Operator : Logic  Inputs=4  AllPortsSameDT=off  OutDataTypeStr=boolean
  Logical Operator{1..2,10,12,14,16,19,21..25,29,33..34} (15 alike) : Logic  Operator=OR  AllPortsSameDT=off  OutDataTypeStr=boolean
  Logical Operator{11,13,15,17,27} (5 alike) : Logic  Operator=NOT  AllPortsSameDT=off  OutDataTypeStr=boolean
  Logical Operator{4,6,8..9,18,20,26,28,30,32,35..36} (12 alike) : Logic  AllPortsSameDT=off  OutDataTypeStr=boolean
  Logical Operator3 : Logic  Inputs=4  AllPortsSameDT=off  OutDataTypeStr=boolean
  Logical Operator5 : Logic  Inputs=4  AllPortsSameDT=off  OutDataTypeStr=boolean
  Logical Operator7 : Logic  Inputs=8  AllPortsSameDT=off  OutDataTypeStr=boolean
  Relational Operator{,1,4,11,13,15} (6 alike) : RelationalOperator  Operator=<=  OutDataTypeStr=boolean  RndMeth=Simplest
  Relational Operator10 : RelationalOperator  Operator=<  OutDataTypeStr=boolean  RndMeth=Simplest
  Relational Operator{2..3,14,16..17} (5 alike) : RelationalOperator  OutDataTypeStr=boolean  RndMeth=Simplest
  Relational Operator8 : RelationalOperator  Operator=<  OutDataTypeStr=boolean  RndMeth=Simplest
  Relational Operator9 : RelationalOperator  Operator=<  OutDataTypeStr=boolean  RndMeth=Simplest
  Subsystem : Subsystem
  Subsystem1 : Subsystem
  Subsystem2 : Subsystem
  Switch{,1..3} (4 alike) : Switch  Criteria=u2 > Threshold
  Terminator_{1..5,9,34..39,54..59} (18 alike) : Terminator
  Unit Delay1 : UnitDelay  SampleTime=-1
  Unit Delay2 : UnitDelay  SampleTime=-1
  Md56MdDone_Val_write : Outport
      settings: EnsureOutportIsVirtual=on
  Md56R2LBkReclinFirstStepPassFlg_Val_write : Outport  Port=2
      settings: EnsureOutportIsVirtual=on
  Md56R2RBkReclinFirstStepPassFlg_Val_write : Outport  Port=3
      settings: EnsureOutportIsVirtual=on
  Md56Stage1DoneResetFlg_Val_write : Outport  Port=4
      settings: EnsureOutportIsVirtual=on
  wires:
  Demux5/3 -> Terminator_35/1
  Md56R2LBkReclnUpwdDnwdTrgtPosCalib1_TrgtPosArray_read/1 -> Demux5/1
  Demux5/2 -> Terminator_36/1
  Demux4/1 -> [Md56R2LBkReclnUpwdDnwdTrgtPos]
  Md56R2LBkReclnUpwdDnwdTrgtPosCalib_TrgtPosArray_read/1 -> Demux4/1
  Demux5/1 -> [Md56R2LBkReclnUpwdDnwdTrgtPos1]
  Demux4/2 -> Terminator_37/1
  Demux4/3 -> Terminator_34/1
  Demux1/1 -> [Md56R2RBkReclnUpwdDnwdTrgtPos]
  Demux1/2 -> Terminator_39/1
  Demux1/3 -> Terminator_38/1
  Md56R2RBkReclnUpwdDnwdTrgtPosCalib_TrgtPosArray_read/1 -> Demux1/1
  Md56R2RBkReclnUpwdDnwdTrgtPosCalib1_TrgtPosArray_read/1 -> Demux2/1
  Demux2/3 -> Terminator_54/1
  Demux2/2 -> Terminator_55/1
  Demux2/1 -> [Md56R2RBkReclnUpwdDnwdTrgtPos1]
  Demux3/1 -> [Md56R3LBkReclnUpwdDnwdTrgtPos]
  Demux3/2 -> Terminator_57/1
  Demux3/3 -> Terminator_56/1
  Md56R3LBkReclnUpwdDnwdTrgtPosCalib_TrgtPosArray_read/1 -> Demux3/1
  Md56R3RBkReclnUpwdDnwdTrgtPosCalib_TrgtPosArray_read/1 -> Demux6/1
  Demux6/3 -> Terminator_58/1
  Demux6/2 -> Terminator_59/1
  Demux6/1 -> [Md56R3RBkReclnUpwdDnwdTrgtPos]
  SecRwRtStLgrstUpwdDnwdStgDone_Val_read/1 -> [SecRwRtStLgrstUpwdDnwdStgDone]
  ThdRwRtStBkReclnStgDone_Val_read/1 -> [ThdRwRtStBkReclnStgDone]
  ThdRwRtStFwdBkwdStgDone_Val_read/1 -> [ThdRwRtStFwdBkwdStgDone]
  ZeroLStgDone_Val_read/1 -> [ZeroLStgDone]
  ThdRwLtStBkReclnStgDone_Val_read/1 -> [ThdRwLtStBkReclnStgDone]
  SecRwLtStFrwdBkwdStgDone_Val_read/1 -> [SecRwLtStFrwdBkwdStgDone]
  SecRwLtStLgrstUpwdDnwdStgDone_Val_read/1 -> [SecRwLtStLgrstUpwdDnwdStgDone]
  ThdRwLtStFwdBkwdStgDone_Val_read/1 -> [ThdRwLtStFwdBkwdStgDone]
  SecRwRtStLgrstOtwdInwdStgDone_Val_read/1 -> [SecRwRtStLgrstOtwdInwdStgDone]
  SecRwLtStLgrstOtwdInwdStgDone_Val_read/1 -> [SecRwLtStLgrstOtwdInwdStgDone]
  SecRwLtStBkReclnStgDone_Val_read/1 -> [SecRwLtStBkReclnStgDone]
  ZeroRStgDone_Val_read/1 -> [ZeroRStgDone]
  ThdRwLtStCshnFldStgDone_Val_read/1 -> [ThdRwLtStCshnFldStgDone]
  SecRwRtStFrwdBkwdStgDone_Val_read/1 -> [SecRwRtStFrwdBkwdStgDone]
  ThdRwRtStCshnFldStgDone_Val_read/1 -> [ThdRwRtStCshnFldStgDone]
  SecRwRtStBkReclnStgDone_Val_read/1 -> [SecRwRtStBkReclnStgDone]
  Constant2/1 -> Switch1/3
  Logical Operator9/1 -> Switch/2
  Constant1/1 -> Switch1/1
  [AllDone] -> Switch1/2
  Constant/1 -> Switch/1
  Switch/1 -> Md56MdDone_Val_write/1
  Switch1/1 -> Switch/3
  [AllDone] -> Logical Operator9/1
  MdXXIsTargetPosZone_Val_read/1 -> 32BitSelector/1(x)
  32BitSelector/1(y) -> Logical Operator9/2
  Logical Operator29/1 -> Logical Operator30/1
  Relational Operator17/1 -> Logical Operator35/1
  Relational Operator4/1 -> Logical Operator28/2
  Relational Operator16/1 -> Logical Operator35/2
  Subsystem/6(R2RFailflg) -> [R2RFailflg]
  [IfVeSMSuThdRwRtStCshnFldUpwdDnwdPos] -> Relational Operator16/1
  [IfVeSMSuSecRwLtStBkReclnUpwdDnwdPos] -> Relational Operator4/1
  If15/1 -> If Action Subsystem26/Action
  Constant11/1 -> Relational Operator14/2
  [Md56R2LBkReclnUpwdDnwdTrgtPos1] -> Relational Operator4/2
  [Md56R2LBkReclnUpwdDnwdTrgtPos] -> Relational Operator13/2
  If13/2 -> If Action Subsystem23/Action
  Logical Operator34/1 -> Logical Operator25/1
  Logical Operator28/1 -> Logical Operator33/2
  [IfVeSMSuSecRwLtStBkReclnUpwdDnwdPos] -> Relational Operator13/1
  Constant8/1 -> Relational Operator9/2
  Logical Operator32/1 -> Logical Operator33/1
  Logical Operator30/1 -> Logical Operator34/1
  Relational Operator14/1 -> Logical Operator32/1
  If12/2 -> If Action Subsystem21/Action
  Subsystem/8(R2RLgrstUpwdDnwdEn) -> If12/1
  [IfVeSMSuSecRwRtStBkReclnUpwdDnwdPos] -> Relational Operator11/1
  [IfVeSMSuThdRwRtStCshnFldUpwdDnwdPos] -> Relational Operator10/1
  Relational Operator9/1 -> Logical Operator29/1
  Relational Operator8/1 -> Logical Operator28/1
  If8/1 -> If Action Subsystem14/Action
  Subsystem/9(R2RZeroEn) -> If13/1
  If9/2 -> If Action Subsystem15/Action
  [Stage1Done] -> Logical Operator5/1
  Constant9/1 -> Relational Operator10/2
  Subsystem/5(R2LBkReclnEn) -> [R2LBkReclinEn], If14/1
  Relational Operator13/1 -> Logical Operator32/2
  Subsystem/4(R2LZeroEn) -> If10/1
  [SecRwLtStBkReclnStgDone] -> Logical Operator24/2
  If12/1 -> If Action Subsystem22/Action
  Subsystem/10(R2RBkReclnEn) -> [R2RBkReclinEn], If15/1
  Subsystem/1(R2LFailflg) -> [R2LFailflg]
  If14/1 -> If Action Subsystem25/Action
  If11/2 -> If Action Subsystem19/Action
  Subsystem/7(R2RLgrstInwdOtwdEn) -> If11/1
  [Md56R2RBkReclnUpwdDnwdTrgtPos] -> Relational Operator15/2
  If8/2 -> If Action Subsystem11/Action
  If10/1 -> If Action Subsystem18/Action
  Subsystem/2(R2LLgrstInwdOtwdEn) -> If8/1
  If10/2 -> If Action Subsystem17/Action
  Constant7/1 -> Relational Operator8/2
  Subsystem/3(R2LLgrstUpwdDnwdEn) -> If9/1
  [SecRwRtStLgrstUpwdDnwdStgDone] -> Subsystem/4(SecRwRtStLgrstUpwdDnwdStgDone_Val_read)
  Logical Operator5/1 -> [AllDone]
  [SecRwLtStLgrstOtwdInwdStgDone] -> Subsystem/1(SecRwLtStLgrstOtwdInwdStgDone_Val_read)
  [SecRwRtStLgrstOtwdInwdStgDone] -> Subsystem/3(SecRwRtStLgrstOtwdInwdStgDone_Val_read)
  [ZeroRStgDone] -> Subsystem/6(ZeroRStgDone_Val_read)
  [Stage2Done] -> Logical Operator5/2
  If11/1 -> If Action Subsystem20/Action
  [ZeroLStgDone] -> Subsystem/5(ZeroLStgDone_Val_read)
  [SecRwRtStBkReclnStgDone] -> Logical Operator25/2
  Constant13/1 -> Relational Operator16/2
  [IfVeSMSuThdRwLtStCshnFldUpwdDnwdPos] -> Relational Operator8/1
  Constant12/1 -> Relational Operator17/2
  Relational Operator11/1 -> Logical Operator30/2
  Relational Operator15/1 -> Logical Operator36/2
  Logical Operator25/1 -> [Stg1R2RBkDone], Subsystem/12(SecRwRtStBkReclnStgDone)
  [SecRwLtStLgrstUpwdDnwdStgDone] -> Subsystem/2(SecRwLtStLgrstUpwdDnwdStgDone_Val_read)
  Logical Operator33/1 -> Logical Operator24/1
  Logical Operator35/1 -> Logical Operator36/1
  If9/1 -> If Action Subsystem16/Action
  Logical Operator24/1 -> [Stg1R2LBkDone], Subsystem/11(SecRwLtStBkReclnStgDone)
  If13/1 -> If Action Subsystem24/Action
  [Md56R2RBkReclnUpwdDnwdTrgtPos1] -> Relational Operator11/2
  Relational Operator10/1 -> Logical Operator29/2
  Logical Operator36/1 -> Logical Operator34/2
  [IfVeSMSuThdRwLtStCshnFldUpwdDnwdPos] -> Relational Operator17/1
  [IfVeSMSuThdRwLtStCshnFldUpwdDnwdPos] -> Relational Operator14/1
  [IfVeSMSuSecRwRtStBkReclnUpwdDnwdPos] -> Relational Operator15/1
  [IfVeSMSuThdRwLtStCshnFldUpwdDnwdPos] -> Relational Operator9/1
  IfVeSMSuThdRwLtStBkReclnUpwdDnwdPos_Val_read/1 -> [IfVeSMSuThdRwLtStBkReclnUpwdDnwdPos]
  IfVeSMSuThdRwRtStBkReclnUpwdDnwdPos_Val_read/1 -> [IfVeSMSuThdRwRtStBkReclnUpwdDnwdPos]
  IfVeSMSuThdRwLtStCshnFldUpwdDnwdPos_Val_read/1 -> [IfVeSMSuThdRwLtStCshnFldUpwdDnwdPos]
  IfVeSMSuThdRwRtStCshnFldUpwdDnwdPos_Val_read/1 -> [IfVeSMSuThdRwRtStCshnFldUpwdDnwdPos]
  IfVeSMSuSecRwLtStBkReclnUpwdDnwdPos_Val_read/1 -> [IfVeSMSuSecRwLtStBkReclnUpwdDnwdPos]
  IfVeSMSuSecRwRtStBkReclnUpwdDnwdPos_Val_read/1 -> [IfVeSMSuSecRwRtStBkReclnUpwdDnwdPos]
  IfVeSMSuSecRwLtStLgrstUpwdDnwdPos_Val_read/1 -> Subsystem/7(IfVeSMSuSecRwLtStLgrstUpwdDnwdPos_Val_read)
  IfVeSMSuSecRwRtStLgrstUpwdDnwdPos_Val_read/1 -> Subsystem/8(IfVeSMSuSecRwRtStLgrstUpwdDnwdPos_Val_read)
  IfVeSMSuSecRwLtStLgrstOtwdInwdPos_Val_read/1 -> Subsystem/9(IfVeSMSuSecRwLtStLgrstOtwdInwdPos_Val_read)
  IfVeSMSuSecRwRtStLgrstOtwdInwdPos_Val_read/1 -> Subsystem/10(IfVeSMSuSecRwRtStLgrstOtwdInwdPos_Val_read)
  IfVeSMSuThdRwLtStCshnFldUpwdDnwdPosV_Val_read/1 -> Terminator_9/1
  IfVeSMSuThdRwRtStCshnFldUpwdDnwdPosV_Val_read/1 -> Terminator_1/1
  StNumFlg_Is4s_read/1 -> Terminator_2/1
  StNumFlg_Is6s_read/1 -> Terminator_3/1
  StNumFlg_Is6s7s_read/1 -> Terminator_4/1
  StNumFlg_Is7s_read/1 -> Terminator_5/1
  If3/1 -> If Action Subsystem5/Action
  Logical Operator14/1 -> Logical Operator15/1
  Chart/5(R3LCshnFldEn) -> If2/1
  [Stage2En] -> Logical Operator12/2
  Logical Operator11/1 -> If Action Subsystem13/Enable
  [R3RBkReclinEn] -> Logical Operator12/1
  Logical Operator17/1 -> Subsystem2/Enable
  [Stage2En] -> Logical Operator14/2
  Logical Operator16/1 -> Logical Operator17/1
  If7/2 -> If Action Subsystem10/Action
  Logical Operator15/1 -> Subsystem1/Enable
  [R2RBkReclinEn] -> Logical Operator16/1
  Logical Operator10/1 -> Logical Operator11/1
  If3/2 -> If Action Subsystem6/Action
  Logical Operator12/1 -> Logical Operator13/1
  If6/1 -> If Action Subsystem12/Action
  If2/1 -> If Action Subsystem3/Action
  Chart/6(R3RCshnFldEn) -> If3/1
  If2/2 -> If Action Subsystem4/Action
  [R3LBkReclinEn] -> Logical Operator10/1
  Chart/10(TrigComfortMd()) -> Subsystem/Trigger
  [Stage2En] -> Logical Operator10/2
  [R2LBkReclinEn] -> Logical Operator14/1
  Logical Operator13/1 -> If Action Subsystem2/Enable
  If1/1 -> If Action Subsystem1/Action
  If7/1 -> If Action Subsystem9/Action
  [Stage2En] -> Logical Operator16/2
  Chart/3(R3LBkReclnEn) -> [R3LBkReclinEn], If6/1
  Chart/4(R3RBkReclnEn) -> [R3RBkReclinEn], If1/1
  Chart/7(Stage2En) -> [Stage2En], If7/1
  [Md56R3RBkReclnUpwdDnwdTrgtPos] -> Relational Operator/2
  [ThdRwLtStFwdBkwdStgDone] -> Logical Operator7/1
  [IfVeSMSuThdRwLtStBkReclnUpwdDnwdPos] -> Relational Operator1/1
  [SecRwRtStFrwdBkwdStgDone] -> Logical Operator7/4
  Logical Operator7/1 -> [Stage2Done]
  [ThdRwRtStCshnFldStgDone] -> Logical Operator2/1
  Logical Operator23/1 -> Logical Operator6/2
  [Stg1R2LBkDone] -> Logical Operator/2
  [IfVeSMSuThdRwRtStBkReclnUpwdDnwdPos] -> Relational Operator/1
  [ThdRwLtStBkReclnStgDone] -> Logical Operator7/5
  [R2LFailflg] -> Logical Operator19/2
  [SecRwRtStLgrstUpwdDnwdStgDone] -> Logical Operator20/2
  Logical Operator18/1 -> Logical Operator19/1
  Relational Operator/1 -> Logical Operator23/1, [FirstStgR3RBkReclnNotMovFlg]
  [Stg1R2RBkDone] -> Logical Operator3/2
  [SecRwRtStBkReclnStgDone] -> Logical Operator7/8
  [SecRwLtStLgrstUpwdDnwdStgDone] -> Logical Operator18/2
  [SecRwLtStBkReclnStgDone] -> Logical Operator7/7
  [Md56R3LBkReclnUpwdDnwdTrgtPos] -> Relational Operator1/2
  [ZeroRStgDone] -> Logical Operator3/4
  [ZeroLStgDone] -> Logical Operator/4
  Logical Operator2/1 -> Logical Operator3/1
  [ThdRwLtStBkReclnStgDone] -> Logical Operator1/2
  [ThdRwLtStCshnFldStgDone] -> Logical Operator22/1
  Logical Operator/1 -> [Stage1LDone]
  Logical Operator6/1 -> Logical Operator2/2
  [ThdRwRtStBkReclnStgDone] -> Logical Operator23/2
  Relational Operator3/1 -> Logical Operator6/1
  [IfVeSMSuThdRwRtStCshnFldUpwdDnwdPos] -> Relational Operator3/1
  [Stage1LDone] -> Logical Operator4/1
  Logical Operator1/1 -> Logical Operator8/2
  Logical Operator22/1 -> Logical Operator/1
  Logical Operator8/1 -> Logical Operator22/2
  Constant4/1 -> Relational Operator3/2
  [Stage1RDone] -> Logical Operator4/2
  Relational Operator1/1 -> [FirstStgR3LBkReclnNotMovFlg], Logical Operator1/1
  Constant3/1 -> Relational Operator2/2
  [SecRwLtStLgrstOtwdInwdStgDone] -> Logical Operator18/1
  Relational Operator2/1 -> Logical Operator8/1
  [SecRwRtStLgrstOtwdInwdStgDone] -> Logical Operator20/1
  Logical Operator20/1 -> Logical Operator21/1
  Logical Operator3/1 -> [Stage1RDone]
  [SecRwLtStFrwdBkwdStgDone] -> Logical Operator7/3
  [ThdRwRtStFwdBkwdStgDone] -> Logical Operator7/2
  Logical Operator21/1 -> Logical Operator3/3
  [R2RFailflg] -> Logical Operator21/2
  Logical Operator19/1 -> Logical Operator/3
  [ThdRwRtStBkReclnStgDone] -> Logical Operator7/6
  [IfVeSMSuThdRwLtStCshnFldUpwdDnwdPos] -> Relational Operator2/1
  FirstTrig/1 -> Switch2/2
  Logical Operator27/1 -> Logical Operator26/2
  Constant5/1 -> Switch2/1
  Switch3/1 -> Switch2/3
  Constant6/1 -> Switch3/1
  Switch2/1 -> [Stage1Done], Logical Operator26/1, Unit Delay2/1
  Unit Delay2/1 -> Logical Operator27/1, Switch3/3
  Unit Delay1/1 -> Switch3/2
  Logical Operator4/1 -> Unit Delay1/1
  Chart/1(R2LBkReclinFirstStepPassFlg) -> Md56R2LBkReclinFirstStepPassFlg_Val_write/1
  Chart/2(R2RBkReclinFirstStepPassFlg) -> Md56R2RBkReclinFirstStepPassFlg_Val_write/1
  Logical Operator26/1 -> Md56Stage1DoneResetFlg_Val_write/1
  [ThdRwLtStBkReclnStgDone] -> Chart/3(ThdRwLtStBkReclnStgDone)
  [ThdRwRtStBkReclnStgDone] -> Chart/4(ThdRwRtStBkReclnStgDone)
  [Md56R2LBkReclnUpwdDnwdTrgtPos1] -> Chart/9(EZER2LBkReclnUpwdDnwdTrgtPos1)
  [Md56R2RBkReclnUpwdDnwdTrgtPos1] -> Chart/10(EZER2RBkReclnUpwdDnwdTrgtPos1)
  [ThdRwRtStCshnFldStgDone] -> Chart/15(ThdRwRtStCshnFldStgDone)
  [Stage2Done] -> Chart/12(Stage2Done)
  [FirstStgR3RBkReclnNotMovFlg] -> Chart/14(FirstStgR3RBkReclnNotMovFlg)
  [FirstStgR3LBkReclnNotMovFlg] -> Chart/13(FirstStgR3LBkReclnNotMovFlg)
  [ThdRwLtStCshnFldStgDone] -> Chart/16(ThdRwLtStCshnFldStgDone)
  [Stage1Done] -> Chart/11(Stage1Done)
  [IfVeSMSuThdRwLtStCshnFldUpwdDnwdPos] -> Chart/5(IfVeSMSuThdRwLtStCshnFldUpwdDnwdPos)
  [IfVeSMSuThdRwRtStCshnFldUpwdDnwdPos] -> Chart/6(IfVeSMSuThdRwRtStCshnFldUpwdDnwdPos)
  [IfVeSMSuSecRwLtStBkReclnUpwdDnwdPos] -> Chart/7(IfVeSMSuSecRwLtStBkReclnUpwdDnwdPos)
  [IfVeSMSuSecRwRtStBkReclnUpwdDnwdPos] -> Chart/8(IfVeSMSuSecRwRtStBkReclnUpwdDnwdPos)
  [Stg1R2RBkDone] -> Chart/17(SecRwRtStBkReclnStgDone)
  [Stg1R2LBkDone] -> Chart/18(SecRwLtStBkReclnStgDone)
  PassStBkReclnStgDone_Val_read/1 -> [PassStBkReclnStgDone]
  PassStFwdBkwdStgDone_Val_read/1 -> [PassStFwdBkwdStgDone]
  [PassStFwdBkwdStgDone] -> Chart/2(PassStFwdBkwdStgDone)
  [PassStBkReclnStgDone] -> Chart/1(PassStBkReclnStgDone)
  If4/2 -> If Action Subsystem27/Action
  If4/1 -> If Action Subsystem7/Action
  Chart/8(PassStFwdBkwdEn) -> If4/1
  If5/2 -> If Action Subsystem28/Action
  If5/1 -> If Action Subsystem8/Action
  Chart/9(PassStBkReclnEn) -> If5/1
  [PassStBkReclnStgDone] -> Logical Operator5/3
  [PassStFwdBkwdStgDone] -> Logical Operator5/4

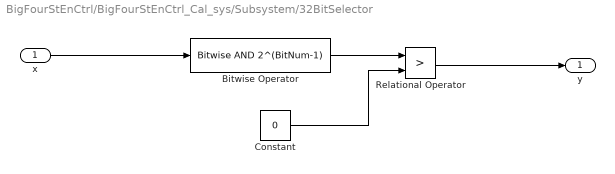
== system BigFourStEnCtrl/BigFourStEnCtrl_Cal_sys/Subsystem/32BitSelector ==
  x : Inport
  Bitwise Operator : simulink/Logic and Bit Operations/Bitwise Operator  logicop=AND  UseBitMask=on  BitMask=2^(BitNum-1)  BitMaskRealWorld=Stored Integer
  Constant : Constant  Value=0  OutDataTypeStr=uint32
  Relational Operator : RelationalOperator  Operator=>  OutDataTypeStr=boolean  RndMeth=Simplest
  y : Outport
  wires:
  Relational Operator/1 -> y/1
  Constant/1 -> Relational Operator/2
  x/1 -> Bitwise Operator/1
  Bitwise Operator/1 -> Relational Operator/1

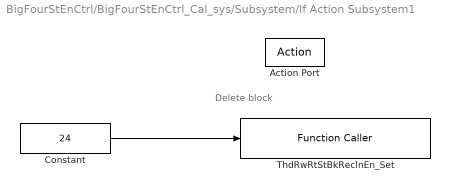
== system BigFourStEnCtrl/BigFourStEnCtrl_Cal_sys/Subsystem/If Action Subsystem1 ==
  note: Delete block
  Action Port : ActionPort  ActionType=then
  Constant : Constant  Value=24  OutDataTypeStr=uint8
  ThdRwRtStBkReclnEn_Set : FunctionCaller  FunctionPrototype=ThdRwRtStBkReclnEn_Set(data)  InputArgumentSpecifications=uint8(1)
  wires:
  Constant/1 -> ThdRwRtStBkReclnEn_Set/1

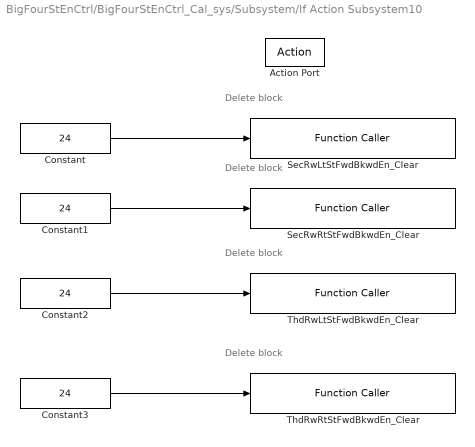
== system BigFourStEnCtrl/BigFourStEnCtrl_Cal_sys/Subsystem/If Action Subsystem10 ==
  note: Delete block
  note: Delete block
  note: Delete block
  note: Delete block
  Action Port : ActionPort  ActionType=else
  Constant{,1..3} (4 alike) : Constant  Value=24  OutDataTypeStr=uint8
  SecRwLtStFwdBkwdEn_Clear : FunctionCaller  FunctionPrototype=SecRwLtStFwdBkwdEn_Clear(data)  InputArgumentSpecifications=uint8(1)
  SecRwRtStFwdBkwdEn_Clear : FunctionCaller  FunctionPrototype=SecRwRtStFwdBkwdEn_Clear(data)  InputArgumentSpecifications=uint8(1)
  ThdRwLtStFwdBkwdEn_Clear : FunctionCaller  FunctionPrototype=ThdRwLtStFwdBkwdEn_Clear(data)  InputArgumentSpecifications=uint8(1)
  ThdRwRtStFwdBkwdEn_Clear : FunctionCaller  FunctionPrototype=ThdRwRtStFwdBkwdEn_Clear(data)  InputArgumentSpecifications=uint8(1)
  wires:
  Constant/1 -> SecRwLtStFwdBkwdEn_Clear/1
  Constant1/1 -> SecRwRtStFwdBkwdEn_Clear/1
  Constant2/1 -> ThdRwLtStFwdBkwdEn_Clear/1
  Constant3/1 -> ThdRwRtStFwdBkwdEn_Clear/1

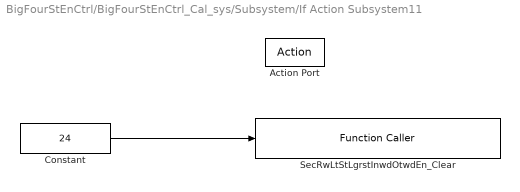
== system BigFourStEnCtrl/BigFourStEnCtrl_Cal_sys/Subsystem/If Action Subsystem11 ==
  Action Port : ActionPort  ActionType=else
  Constant : Constant  Value=24  OutDataTypeStr=uint8
  SecRwLtStLgrstInwdOtwdEn_Clear : FunctionCaller  FunctionPrototype=SecRwLtStLgrstInwdOtwdEn_Clear(data)  InputArgumentSpecifications=uint8(1)
  wires:
  Constant/1 -> SecRwLtStLgrstInwdOtwdEn_Clear/1

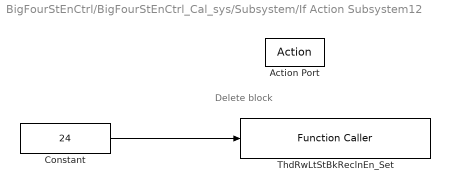
== system BigFourStEnCtrl/BigFourStEnCtrl_Cal_sys/Subsystem/If Action Subsystem12 ==
  note: Delete block
  Action Port : ActionPort  ActionType=then
  Constant : Constant  Value=24  OutDataTypeStr=uint8
  ThdRwLtStBkReclnEn_Set : FunctionCaller  FunctionPrototype=ThdRwLtStBkReclnEn_Set(data)  InputArgumentSpecifications=uint8(1)
  wires:
  Constant/1 -> ThdRwLtStBkReclnEn_Set/1

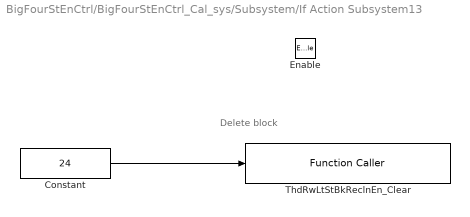
== system BigFourStEnCtrl/BigFourStEnCtrl_Cal_sys/Subsystem/If Action Subsystem13 ==
  note: Delete block
  Enable : EnablePort
  Constant : Constant  Value=24  OutDataTypeStr=uint8
  ThdRwLtStBkReclnEn_Clear : FunctionCaller  FunctionPrototype=ThdRwLtStBkReclnEn_Clear(data)  InputArgumentSpecifications=uint8(1)
  wires:
  Constant/1 -> ThdRwLtStBkReclnEn_Clear/1

== system BigFourStEnCtrl/BigFourStEnCtrl_Cal_sys/Subsystem/If Action Subsystem14 ==
  Action Port : ActionPort  ActionType=then
  Constant : Constant  Value=24  OutDataTypeStr=uint8
  SecRwLtStLgrstInwdOtwdEn_Set : FunctionCaller  FunctionPrototype=SecRwLtStLgrstInwdOtwdEn_Set(data)  InputArgumentSpecifications=uint8(1)
  wires:
  Constant/1 -> SecRwLtStLgrstInwdOtwdEn_Set/1

== system BigFourStEnCtrl/BigFourStEnCtrl_Cal_sys/Subsystem/If Action Subsystem15 ==
  Action Port : ActionPort  ActionType=else
  Constant : Constant  Value=24  OutDataTypeStr=uint8
  SecRwLtStLgrstUpwdDnwdEn_Clear : FunctionCaller  FunctionPrototype=SecRwLtStLgrstUpwdDnwdEn_Clear(data)  InputArgumentSpecifications=uint8(1)
  wires:
  Constant/1 -> SecRwLtStLgrstUpwdDnwdEn_Clear/1

== system BigFourStEnCtrl/BigFourStEnCtrl_Cal_sys/Subsystem/If Action Subsystem16 ==
  Action Port : ActionPort  ActionType=then
  Constant : Constant  Value=24  OutDataTypeStr=uint8
  SecRwLtStLgrstUpwdDnwdEn_Set : FunctionCaller  FunctionPrototype=SecRwLtStLgrstUpwdDnwdEn_Set(data)  InputArgumentSpecifications=uint8(1)
  wires:
  Constant/1 -> SecRwLtStLgrstUpwdDnwdEn_Set/1

== system BigFourStEnCtrl/BigFourStEnCtrl_Cal_sys/Subsystem/If Action Subsystem17 ==
  Action Port : ActionPort  ActionType=else
  Constant : Constant  Value=24  OutDataTypeStr=uint8
  ZeroLEn_Clear : FunctionCaller  FunctionPrototype=ZeroLEn_Clear(data)  InputArgumentSpecifications=uint8(1)
  wires:
  Constant/1 -> ZeroLEn_Clear/1

== system BigFourStEnCtrl/BigFourStEnCtrl_Cal_sys/Subsystem/If Action Subsystem18 ==
  Action Port : ActionPort  ActionType=then
  Constant : Constant  Value=24  OutDataTypeStr=uint8
  ZeroLEn_Set : FunctionCaller  FunctionPrototype=ZeroLEn_Set(data)  InputArgumentSpecifications=uint8(1)
  wires:
  Constant/1 -> ZeroLEn_Set/1

== system BigFourStEnCtrl/BigFourStEnCtrl_Cal_sys/Subsystem/If Action Subsystem19 ==
  Action Port : ActionPort  ActionType=else
  Constant : Constant  Value=24  OutDataTypeStr=uint8
  SecRwRtStLgrstInwdOtwdEn_Clear : FunctionCaller  FunctionPrototype=SecRwRtStLgrstInwdOtwdEn_Clear(data)  InputArgumentSpecifications=uint8(1)
  wires:
  Constant/1 -> SecRwRtStLgrstInwdOtwdEn_Clear/1

== system BigFourStEnCtrl/BigFourStEnCtrl_Cal_sys/Subsystem/If Action Subsystem2 ==
  note: Delete block
  Enable : EnablePort
  Constant : Constant  Value=24  OutDataTypeStr=uint8
  ThdRwRtStBkReclnEn_Clear : FunctionCaller  FunctionPrototype=ThdRwRtStBkReclnEn_Clear(data)  InputArgumentSpecifications=uint8(1)
  wires:
  Constant/1 -> ThdRwRtStBkReclnEn_Clear/1

== system BigFourStEnCtrl/BigFourStEnCtrl_Cal_sys/Subsystem/If Action Subsystem20 ==
  Action Port : ActionPort  ActionType=then
  Constant : Constant  Value=24  OutDataTypeStr=uint8
  SecRwRtStLgrstInwdOtwdEn_Set : FunctionCaller  FunctionPrototype=SecRwRtStLgrstInwdOtwdEn_Set(data)  InputArgumentSpecifications=uint8(1)
  wires:
  Constant/1 -> SecRwRtStLgrstInwdOtwdEn_Set/1

== system BigFourStEnCtrl/BigFourStEnCtrl_Cal_sys/Subsystem/If Action Subsystem21 ==
  Action Port : ActionPort  ActionType=else
  Constant : Constant  Value=24  OutDataTypeStr=uint8
  SecRwRtStLgrstUpwdDnwdEn_Clear : FunctionCaller  FunctionPrototype=SecRwRtStLgrstUpwdDnwdEn_Clear(data)  InputArgumentSpecifications=uint8(1)
  wires:
  Constant/1 -> SecRwRtStLgrstUpwdDnwdEn_Clear/1

== system BigFourStEnCtrl/BigFourStEnCtrl_Cal_sys/Subsystem/If Action Subsystem22 ==
  Action Port : ActionPort  ActionType=then
  Constant : Constant  Value=24  OutDataTypeStr=uint8
  SecRwRtStLgrstUpwdDnwdEn_Set : FunctionCaller  FunctionPrototype=SecRwRtStLgrstUpwdDnwdEn_Set(data)  InputArgumentSpecifications=uint8(1)
  wires:
  Constant/1 -> SecRwRtStLgrstUpwdDnwdEn_Set/1

== system BigFourStEnCtrl/BigFourStEnCtrl_Cal_sys/Subsystem/If Action Subsystem23 ==
  Action Port : ActionPort  ActionType=else
  Constant : Constant  Value=24  OutDataTypeStr=uint8
  ZeroREn_Clear : FunctionCaller  FunctionPrototype=ZeroREn_Clear(data)  InputArgumentSpecifications=uint8(1)
  wires:
  Constant/1 -> ZeroREn_Clear/1

== system BigFourStEnCtrl/BigFourStEnCtrl_Cal_sys/Subsystem/If Action Subsystem24 ==
  Action Port : ActionPort  ActionType=then
  Constant : Constant  Value=24  OutDataTypeStr=uint8
  ZeroREn_Set : FunctionCaller  FunctionPrototype=ZeroREn_Set(data)  InputArgumentSpecifications=uint8(1)
  wires:
  Constant/1 -> ZeroREn_Set/1

== system BigFourStEnCtrl/BigFourStEnCtrl_Cal_sys/Subsystem/If Action Subsystem25 ==
  note: Delete block
  Action Port : ActionPort  ActionType=then
  Constant : Constant  Value=24  OutDataTypeStr=uint8
  SecRwLtStBkReclnEn_Set : FunctionCaller  FunctionPrototype=SecRwLtStBkReclnEn_Set(data)  InputArgumentSpecifications=uint8(1)
  wires:
  Constant/1 -> SecRwLtStBkReclnEn_Set/1
